simulink model "sl_aerialmanipulator"  (R2016b)
settings: Solver=FixedStepAuto  StartTime=0.0  StopTime=20  RelTol=1e-3
InitFcn:
  | % load a dynamic model of the quadrotor
  | mdl_aerialmanipulator
values from neighbouring files (symbols this model uses):
  ps = cam.project(Marker, 'Tcam', transl(CenterBias'+[0 0 TargetHeight])*trotx(-pi))    [mdl_aerialmanipulator.m]
undefined symbols (not defined in the file or in its folder): aerialmanipulator, rpy2tr, transl
undefined symbols (not defined in the file): manipulator
libraries: roblocks x6
settings Model: Creator=zhonghang  LastModifiedBy=dell
settings SolverCC: ZeroCrossControl=EnableAll
settings DataIOCC: LimitDataPoints=on  SaveFormat=Array
settings OptimizationCC: DefaultParameterBehavior=Inlined  UseDivisionForNetSlopeComputation=on  UseFloatMulNetSlope=on  InlineInvariantSignals=on  PassReuseOutputArgsAs=Individual arguments  ZeroExternalMemoryAtStartup=off  ZeroInternalMemoryAtStartup=off  NoFixptDivByZeroProtection=on  EfficientFloat2IntCast=on  LifeSpan=1
settings DebuggingCC: ParameterTunabilityLossMsg=error  SFUnexpectedBacktrackingDiag=warning  SFNoUnconditionalDefaultTransitionDiag=warning  SFExecutionAtInitializationDiag=none
settings ModelReferenceCC: PropagateSignalLabelsOutOfModel=off
settings RTWCC: SystemTargetFile=ert.tlc  TemplateMakefile=ert_default_tmf  Description=Embedded Coder  GenerateReport=on  IncludeHyperlinkInReport=on  LaunchReport=on  GenerateTraceInfo=on  GenerateTraceReport=on  GenerateTraceReportSl=on  GenerateTraceReportSf=on  GenerateTraceReportEml=on  GenerateCodeMetricsReport=on
settings CodeAppCC: ForceParamTrailComments=on  IgnoreCustomStorageClasses=off  OperatorAnnotations=on  SimulinkDataObjDesc=on  SFDataObjDesc=on  MATLABFcnDesc=on  CustomSymbolStrGlobalVar=rt$N$M  CustomSymbolStrType=$N$M  CustomSymbolStrFcn=$N$M$F  CustomSymbolStrMacro=$N$M  InsertBlockDesc=on  MATLABSourceComments=on
settings ERTTargetCC: GenerateSampleERTMain=on  CombineSignalStateStructs=on  SupportAbsoluteTime=off  SupportComplex=off  SupportContinuousTime=on  SupportNonInlinedSFcns=on  InlinedParameterPlacement=NonHierarchical  ERTCustomFileTemplate=example_file_process.tlc  ERTFilePackagingFormat=CompactWithDataFile
settings ConfigComp: CovMetricSettings=dw  CovHtmlReporting=on  CovSaveCumulativeToWorkspaceVar=on  CovSaveSingleToWorkspaceVar=on  CovExternalEMLEnable=off

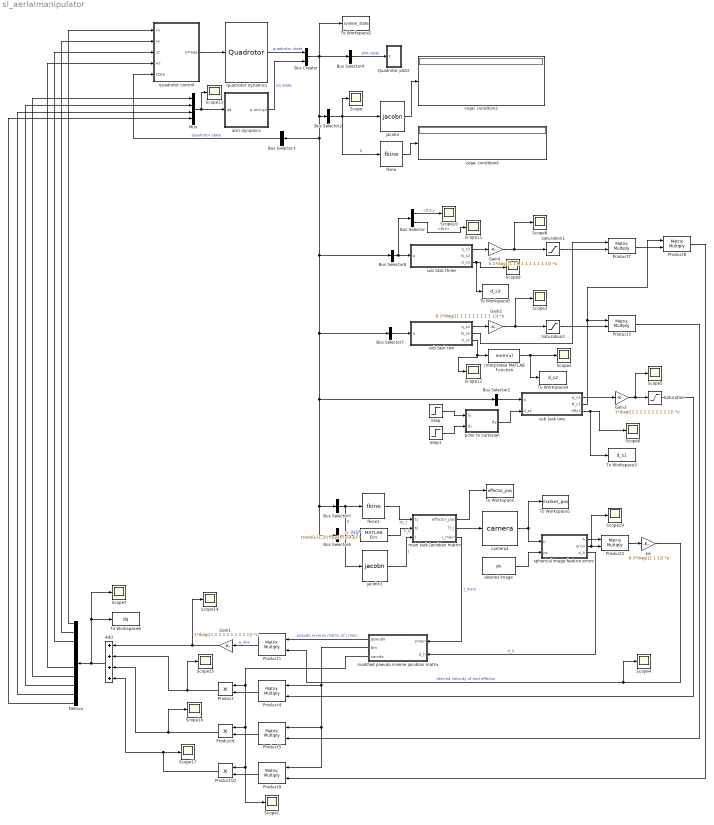
== system sl_aerialmanipulator ==
  -> SE2 : MATLABFcn  MATLABFcn=transl(u(1:3))*rpy2tr(u(4:6)')  OutputDimensions=[4 4]  Output1D=off
  Add : Sum  Inputs=++++
  Bus Creator : BusCreator  Inputs=2
  Bus Selector : BusSelector  OutputSignals=th1,th4
  Bus Selector1 : BusSelector  OutputSignals=quadrotor state.X,quadrotor state.Y,quadrotor state.Z,quadrotor state.roll,quadrotor state.pitch,quadrotor state.yaw,rm state.th1,rm state.th2,rm state.th3,rm state.th4  OutputAsBus=on
  Bus Selector{2,5,7..8} (4 alike) : BusSelector  OutputSignals=rm state.th1,rm state.th2,rm state.th3,rm state.th4  OutputAsBus=on
  Bus Selector3 : BusSelector  OutputSignals=quadrotor state.X,quadrotor state.Y,quadrotor state.Z,quadrotor state.yaw,quadrotor state.pitch,quadrotor state.roll,quadrotor state.dx,quadrotor state.dy,quadrotor state.dz,quadrotor state.dyaw,quadrotor state.dpitch,quadrotor state.droll  OutputAsBus=on
  Bus Selector4 : BusSelector  OutputSignals=quadrotor state.X,quadrotor state.Y,quadrotor state.Z,quadrotor state.yaw,quadrotor state.pitch,quadrotor state.roll,rm state.th1,rm state.th2,rm state.th3,rm state.th4  OutputAsBus=on
  Bus Selector6 : BusSelector  OutputSignals=quadrotor state.X,quadrotor state.Y,quadrotor state.Z,quadrotor state.yaw,quadrotor state.pitch,quadrotor state.roll  OutputAsBus=on
  Demux : Demux  Outputs=10
  Gain1 : Gain  Gain=1*diag([1 1 1 1 1 1 1 1 1 1])  Multiplication=Matrix(K*u)
  Gain2 : Gain  Gain=-0.1*diag([1 1 1 1 1 1 1 1 1 1])  Multiplication=Matrix(K*u)
  Gain3 : Gain  Gain=1*diag([1 1 1 1 1 1 1 1 1 1])  Multiplication=Matrix(K*u)
  Gain4 : Gain  Gain=0.1*diag([1 1 1 1 1 1 1 1 1 1])  Multiplication=Matrix(K*u)
  Interpreted MATLAB Function : MATLABFcn  MATLABFcn=norm(u)
  Mux : Mux
  Product : Product
  Product{1..5,7..9} (8 alike) : Product  Multiplication=Matrix(*)
  Product10 : Product
  Product6 : Product
  Quadrotor plot2 : Subsystem  AncestorBlock=roblocks/Robot Graphics/Quadrotor plot  mask{quad=aerialmanipulator, xydim=1.5, zdim=2.5}
      mask prompts: quad "Model"; xydim "xy-axes dimension"; zdim "z-axis dimension"
      mask help: Animate quadrotor.
      mask Help:
      | This block graphically displays a quadrotor (flying robot).
      | 
      | A new figure is created and A graphical model of a quadrotor is animated
      | to a pose specified by the state vector input to the block.
      | 
      | The state vector is [x y z roll pitch yaw] in world coordinates and the
      | angles are in radians.
      | 
      | Notes:
      | - The dimensions of the vehicle workspace are set by parameters
  Saturation : Saturate  UpperLimit=1  LowerLimit=-1
  Saturation1 : Saturate  UpperLimit=1  LowerLimit=-1
  Saturation2 : Saturate  UpperLimit=1  LowerLimit=-1
  Scope{,1..17,19} (19 alike) : Scope
  Step : Step  Time=15  Before=180*pi/180  After=120*pi/180  SampleTime=0
  Step1 : Step  Time=15  Before=0*pi/180  After=-120*pi/180  SampleTime=0
  To Workspace : ToWorkspace  VariableName=effector_pos  SaveFormat=Structure With Time  SampleTime=-1
  To Workspace1 : ToWorkspace  VariableName=marker_pos  SaveFormat=Structure With Time  SampleTime=-1
  To Workspace2 : ToWorkspace  VariableName=system_state  SaveFormat=Structure With Time  SampleTime=-1
  To Workspace3 : ToWorkspace  VariableName=d_s1  SaveFormat=Structure With Time  SampleTime=-1
  To Workspace4 : ToWorkspace  VariableName=d_s2  SaveFormat=Structure With Time  SampleTime=-1
  To Workspace5 : ToWorkspace  VariableName=d_s3  SaveFormat=Structure With Time  SampleTime=-1
  To Workspace6 : ToWorkspace  VariableName=dq  SaveFormat=Structure With Time  SampleTime=-1
  arm dynamics : Subsystem  mask{robotarm=manipulator, q0=[-pi/3 3*pi/4 0 0]}
      mask prompts: robotarm "robot arm object"; q0 "joint initial value"
  camera2 : roblocks/Vision/camera  cam=cam  points=Marker
  desired image : Constant  Value=ps  VectorParams1D=off
  fkine : roblocks/Kinematics/fkine  robot=manipulator
  fkine1 : roblocks/Kinematics/fkine  robot=manipulator
  jacobn : roblocks/Kinematics/jacobn  robot=manipulator
  jacobn1 : roblocks/Kinematics/jacobn  robot=manipulator
  kd : Gain  Gain=0.3*diag([1 1 1])  Multiplication=Matrix(K*u)
  main task Jacobian matrix : MATLAB Function  TreatAsAtomicUnit=on
  modified pseudo inverse jacobian matrix : MATLAB Function  TreatAsAtomicUnit=on
  polor to cartesian : MATLAB Function  TreatAsAtomicUnit=on
  quadrotor control : Subsystem
  quadrotor dynamics : roblocks/Dynamics/Quadrotor  quad=aerialmanipulator
      link override Dynamics: FunctionName=aerialmanipulator_dynamics
  "spherical image feature errors " : MATLAB Function  TreatAsAtomicUnit=on
  sub task one : MATLAB Function  TreatAsAtomicUnit=on
  sub task three : MATLAB Function  TreatAsAtomicUnit=on
  sub task two : MATLAB Function  TreatAsAtomicUnit=on
  visjac condition2 : Display
  visjac condition6 : Display
  wires:
  quadrotor control/1(omega) -> quadrotor dynamics/1
  quadrotor dynamics/1 -> Bus Creator/1  "quadrotor state"
  jacobn/1 -> visjac condition2/1
  Bus Selector2/1 -> Scope/1, fkine/1, jacobn/1  "q"
  Bus Selector3/1 -> quadrotor control/5(state)  "quadrotor state"
  Bus Selector4/1 -> Quadrotor plot2/1(X)  "plot state"
  fkine/1 -> visjac condition6/1
  Bus Selector5/1 -> jacobn1/1, fkine1/1  "q"
  Bus Selector6/1 -> -> SE2/1  "quad"
  fkine1/1 -> main task Jacobian matrix/1(t1)  "Tb_t"
  -> SE2/1 -> main task Jacobian matrix/2(t2)  "Ti_b"
  jacobn1/1 -> main task Jacobian matrix/3(J)  "J"
  Product1/1 -> Gain1/1  "q_des"
  "spherical image feature errors "/1(A) -> Product2/1
  Product2/1 -> kd/1
  "spherical image feature errors "/2(error) -> Scope19/1, Product2/2
  "spherical image feature errors "/3(d_h) -> modified pseudo inverse jacobian matrix/2(d_h)  "d_h"
  modified pseudo inverse jacobian matrix/1(Jpseudo) -> Product1/1  "pseudo inverse matrix of J main"
  Bus Selector1/1 -> sub task one/1(q)
  sub task one/1(q_s1) -> Gain3/1
  modified pseudo inverse jacobian matrix/2(Nm) -> Product9/1, Product5/1, Product4/1
  camera2/1 -> "spherical image feature errors "/1(p), To Workspace1/1
  Bus Creator/1 -> To Workspace2/1, Bus Selector3/1, Bus Selector6/1, Bus Selector5/1, Bus Selector1/1, Bus Selector7/1, Bus Selector8/1, Bus Selector2/1, Bus Selector4/1
  Bus Selector7/1 -> sub task two/1(q)
  sub task two/1(q_s2) -> Gain2/1
  Interpreted MATLAB Function/1 -> To Workspace4/1, Scope2/1
  sub task two/3(d_s2) -> Scope12/1, Interpreted MATLAB Function/1
  kd/1 -> Scope4/1, Product1/2  "desired velocity of end effector"
  Gain2/1 -> Saturation2/1, Scope3/1
  sub task one/2(N_s1) -> Product8/1, Product3/1
  Gain3/1 -> Saturation/1, Scope5/1
  Product4/1 -> Product/2
  Product5/1 -> Product6/2
  Bus Selector8/1 -> Bus Selector/1, sub task three/1(q)
  sub task three/1(q_s3) -> Gain4/1
  Gain4/1 -> Saturation1/1, Scope8/1
  Product9/1 -> Product10/2
  sub task three/3(d_s3) -> To Workspace5/1, Scope9/1
  Bus Selector/1 -> Scope10/1  "<th1>"
  Bus Selector/2 -> Scope11/1  "<th4>"
  Gain1/1 -> Scope14/1, Add/1
  Add/1 -> To Workspace6/1, Scope7/1, Demux/1
  Demux/1 -> quadrotor control/1(vx)
  Demux/2 -> quadrotor control/2(vy)
  Demux/3 -> quadrotor control/3(vz)
  Demux/7 -> Mux/1
  Demux/8 -> Mux/2
  Demux/9 -> Mux/3
  main task Jacobian matrix/2(Tt_i) -> camera2/1
  main task Jacobian matrix/3(J_main) -> modified pseudo inverse jacobian matrix/1(Jmain)  "J_main"
  modified pseudo inverse jacobian matrix/3(namda) -> Product6/1, Product10/1, Scope1/1, Product/1
  desired image/1 -> "spherical image feature errors "/2(ps)
  polor to cartesian/1(dy) -> sub task one/2(d_s1)
  Step/1 -> polor to cartesian/1(fy)
  Step1/1 -> polor to cartesian/2(th)
  main task Jacobian matrix/1(effector_pos) -> To Workspace/1
  Saturation2/1 -> Product3/2
  sub task two/2(N_s2) -> Product7/1
  Product7/1 -> Product8/2
  Product/1 -> Add/2, Scope15/1
  Product6/1 -> Add/3, Scope16/1
  Saturation1/1 -> Product7/2
  Product10/1 -> Add/4, Scope17/1
  Saturation/1 -> Product4/2
  Product3/1 -> Product5/2
  Product8/1 -> Product9/2
  sub task one/3(dRs1) -> To Workspace3/1, Scope6/1
  Mux/1 -> Scope13/1, arm dynamics/1(qd)
  arm dynamics/1(q and qd) -> Bus Creator/2  "rm state"
  Demux/6 -> quadrotor control/4(wz)
  Demux/10 -> Mux/4

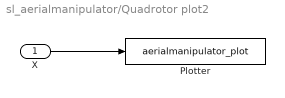
== system sl_aerialmanipulator/Quadrotor plot2 ==
  X : Inport
  Plotter : S-Function  FunctionName=aerialmanipulator_plot  Parameters=[xydim, zdim], 1, 1,aerialmanipulator  SFunctionDeploymentMode=off  EnableBusSupport=off
  wires:
  X/1 -> Plotter/1

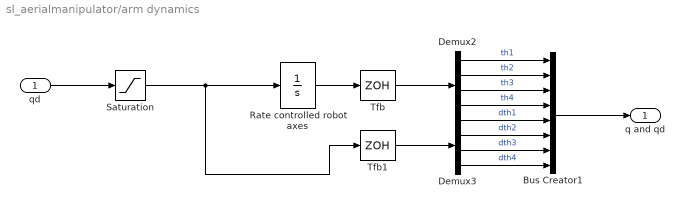
== system sl_aerialmanipulator/arm dynamics ==
  qd : Inport
  Bus Creator1 : BusCreator  Inputs=8
  Demux2 : Demux
  Demux3 : Demux
  Rate controlled robot axes : Integrator  InitialCondition=q0
  Saturation : Saturate  UpperLimit=1  LowerLimit=-1
  Tfb : ZeroOrderHold  SampleTime=0.01
  Tfb1 : ZeroOrderHold  SampleTime=0.01
  q and qd : Outport
  wires:
  qd/1 -> Saturation/1
  Rate controlled robot axes/1 -> Tfb/1
  Demux3/4 -> Bus Creator1/8  "dth4"
  Demux3/3 -> Bus Creator1/7  "dth3"
  Demux3/2 -> Bus Creator1/6  "dth2"
  Demux3/1 -> Bus Creator1/5  "dth1"
  Demux2/4 -> Bus Creator1/4  "th4"
  Demux2/3 -> Bus Creator1/3  "th3"
  Demux2/2 -> Bus Creator1/2  "th2"
  Demux2/1 -> Bus Creator1/1  "th1"
  Bus Creator1/1 -> q and qd/1
  Saturation/1 -> Tfb1/1, Rate controlled robot axes/1
  Tfb/1 -> Demux2/1
  Tfb1/1 -> Demux3/1

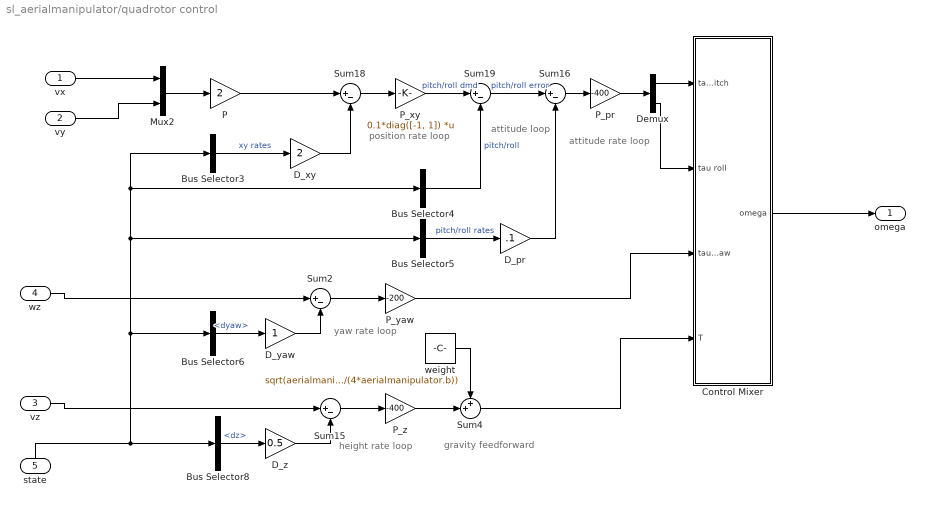
== system sl_aerialmanipulator/quadrotor control ==
  note: gravity feedforward
  note: attitude rate
      | loop
  note: attitude
      | loop
  note: position rate
      | loop
  note: yaw rate
      | loop
  note: height rate
      | loop
  vx : Inport
  vy : Inport  Port=2
  vz : Inport  Port=3
  wz : Inport  Port=4
  state : Inport  Port=5
  Bus Selector3 : BusSelector  OutputSignals=dx,dy  OutputAsBus=on
  Bus Selector4 : BusSelector  OutputSignals=pitch,roll  OutputAsBus=on
  Bus Selector5 : BusSelector  OutputSignals=dpitch,droll  OutputAsBus=on
  Bus Selector6 : BusSelector  OutputSignals=dyaw
  Bus Selector8 : BusSelector  OutputSignals=dz
  Control Mixer : Subsystem  AncestorBlock=roblocks/Dynamics/Control Mixer 4
      mask help: Quadrotor control mixer
      mask Help:
      | Determine rotor speeds based on desired torques and thrust.
      | 
      | <b>Inputs::</b>
      | 
      | tau pitch (1x1)  desired pitching torque [Nm]
      | tau roll (1x1)   desired rolling torque [Nm]
      | tau yaw (1x1)    desired yawing torque [Nm]
      | T (1x1)          desired thrust [N]
      | 
      | <b>Outputs::</b>
      | 
      | w1 (1x1) angular velocity of rotor 1 [rad]
      | w2 (1x1) angular velocity of rotor 2 [rad]
      | w3 (1x1) angular velocity of rotor 3 [rad]
      | w4 (1x1) angular velocity of rotor 4 [rad]
      | 
      | <b>Notes::</b>
      | 
      | - Assumes the rotor labelling convention of RVC Fig 4.16.
      | - The quadrotor is underactuated and has only 4 inputs.
  D_pr : Gain  Gain=.1
  D_xy : Gain  Gain=2
  D_yaw : Gain
  D_z : Gain  Gain=0.5
  Demux : Demux  Outputs=2
  Mux2 : Mux  Inputs=2
  P : Gain  Gain=2
  P_pr : Gain  Gain=-400
  P_xy : Gain  Gain=0.1*diag([-1, 1])  Multiplication=Matrix(K*u)
  P_yaw : Gain  Gain=-200
  P_z : Gain  Gain=-400
  Sum{2,15..16,18..19} (5 alike) : Sum  Inputs=|+-
  Sum4 : Sum  Inputs=++|
  weight : Constant  Value=sqrt(aerialmanipulator.M*aerialmanipulator.g/(4*aerialmanipulator.b))  SampleTime=0
  omega : Outport
  wires:
  state/1 -> Bus Selector8/1, Bus Selector5/1, Bus Selector4/1, Bus Selector3/1, Bus Selector6/1
  Mux2/1 -> P/1
  P/1 -> Sum18/1
  Sum18/1 -> P_xy/1
  wz/1 -> Sum2/1
  vz/1 -> Sum15/1
  Control Mixer/1(omega) -> omega/1
  Bus Selector3/1 -> D_xy/1  "xy rates"
  D_xy/1 -> Sum18/2
  P_xy/1 -> Sum19/1  "pitch/roll dmd"
  Bus Selector4/1 -> Sum19/2  "pitch/roll"
  Sum19/1 -> Sum16/1  "pitch/roll error"
  P_pr/1 -> Demux/1
  Bus Selector6/1 -> D_yaw/1  "<dyaw>"
  Bus Selector8/1 -> D_z/1  "<dz>"
  D_z/1 -> Sum15/2
  D_pr/1 -> Sum16/2
  Demux/2 -> Control Mixer/2(tau roll)
  Sum2/1 -> P_yaw/1
  P_yaw/1 -> Control Mixer/3(tau yaw)
  Demux/1 -> Control Mixer/1(tau pitch)
  Bus Selector5/1 -> D_pr/1  "pitch/roll rates"
  D_yaw/1 -> Sum2/2
  weight/1 -> Sum4/1
  Sum4/1 -> Control Mixer/4(T)
  vx/1 -> Mux2/1
  Sum16/1 -> P_pr/1
  vy/1 -> Mux2/2
  Sum15/1 -> P_z/1
  P_z/1 -> Sum4/2

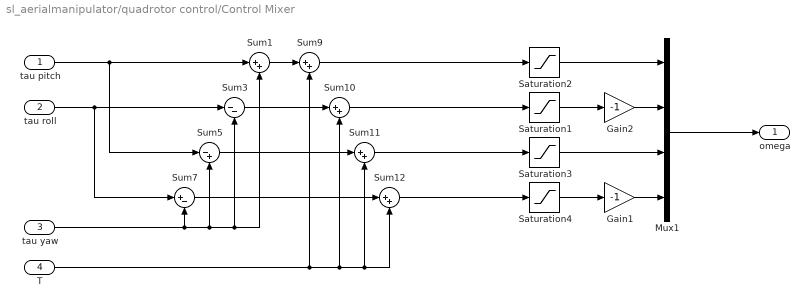
== system sl_aerialmanipulator/quadrotor control/Control Mixer ==
  tau pitch : Inport
  tau roll : Inport  Port=2
  tau yaw : Inport  Port=3
  T : Inport  Port=4
  Gain1 : Gain  Gain=-1
  Gain2 : Gain  Gain=-1
  Mux1 : Mux
  Saturation{1..4} (4 alike) : Saturate  UpperLimit=1000  LowerLimit=700
  Sum{1,9..12} (5 alike) : Sum  Inputs=|++  SaturateOnIntegerOverflow=on  InputSameDT=on  OutDataTypeStr=Inherit: Same as first input
  Sum3 : Sum  Inputs=|--  SaturateOnIntegerOverflow=on  InputSameDT=on  OutDataTypeStr=Inherit: Same as first input
  Sum5 : Sum  Inputs=|-+  SaturateOnIntegerOverflow=on  InputSameDT=on  OutDataTypeStr=Inherit: Same as first input
  Sum7 : Sum  Inputs=|+-  SaturateOnIntegerOverflow=on  InputSameDT=on  OutDataTypeStr=Inherit: Same as first input
  omega : Outport
  wires:
  Mux1/1 -> omega/1
  Gain2/1 -> Mux1/2
  tau yaw/1 -> Sum7/2, Sum5/2, Sum3/2, Sum1/2
  Saturation2/1 -> Mux1/1
  Saturation1/1 -> Gain2/1
  Saturation3/1 -> Mux1/3
  Saturation4/1 -> Gain1/1
  tau pitch/1 -> Sum1/1, Sum5/1
  Sum1/1 -> Sum9/1
  Sum3/1 -> Sum10/1
  Sum5/1 -> Sum11/1
  Sum7/1 -> Sum12/1
  Sum9/1 -> Saturation2/1
  Sum10/1 -> Saturation1/1
  Sum11/1 -> Saturation3/1
  Sum12/1 -> Saturation4/1
  T/1 -> Sum11/2, Sum12/2, Sum10/2, Sum9/2
  tau roll/1 -> Sum3/1, Sum7/1
  Gain1/1 -> Mux1/4

== matlab function sl_aerialmanipulator/main task Jacobian matrix ==
  data: effector_pos output; Tt_i output; t1 input; J_main output; t2 input; J input
function [effector_pos, Tt_i,J_main] = JmainCal(t1, t2, J)
%#codegen

Base_T =[0.7071 0.7071 0 0; ...
    -0.7071 0.7071 0 0; ...
    0 0 -1.0000 0; ...
    0 0 0 1.0000];
s = t2*Base_T*t1;
s1 = s(1:3, 1:3);
% transfer end effevtor to interial coor matrix 
Tt_i = s;
% end effector position
effector_pos = s(1:3,4)';
% R is tthe R_I_T
R = pinv(s1);
% J_l
Jl = J(1:3, :);
% J main task jacobian matrix
J_main = [R zeros(3) Jl];

== matlab function sl_aerialmanipulator/sub task one ==
  data: q_s1 output; N_s1 output; q input; d_s1 input; dRs1 output
function [q_s1, N_s1, dRs1] = SubTskOneJaco(q, d_s1)
%#codegen
%%
x = zeros(10,1);
x = q;
roll = x(4); pitch = x(5); yaw = x(6);
th1 = x(7); th2 = x(8); th3 = x(9); th4 = x(10);
%% jacobian matrix
d_Rs1 = [0, 0, 0, 0, 0, 0,                                                                                                         ((7071*cos(pitch))/10000 + (7071*sin(pitch)*sin(roll))/10000)*((4967757600021511*sin(th1))/81129638414606681695789005144064 + cos(th3)*(cos(th1)*cos(th2) - (4967757600021511*sin(th1)*sin(th2))/81129638414606681695789005144064) - sin(th3)*(cos(th1)*sin(th2) + (4967757600021511*cos(th2)*sin(th1))/81129638414606681695789005144064)) - ((7071*cos(pitch))/10000 - (7071*sin(pitch)*sin(roll))/10000)*(cos(th3)*((4967757600021511*cos(th1)*sin(th2))/81129638414606681695789005144064 + cos(th2)*sin(th1)) - (4967757600021511*cos(th1))/81129638414606681695789005144064 + sin(th3)*((4967757600021511*cos(th1)*cos(th2))/81129638414606681695789005144064 - sin(th1)*sin(th2))),                                                                                                                                         (cos(th3)*((4967757600021511*cos(th1)*cos(th2))/81129638414606681695789005144064 - sin(th1)*sin(th2)) - sin(th3)*((4967757600021511*cos(th1)*sin(th2))/81129638414606681695789005144064 + cos(th2)*sin(th1)))*((7071*cos(pitch))/10000 + (7071*sin(pitch)*sin(roll))/10000) - (cos(th3)*(cos(th1)*sin(th2) + (4967757600021511*cos(th2)*sin(th1))/81129638414606681695789005144064) + sin(th3)*(cos(th1)*cos(th2) - (4967757600021511*sin(th1)*sin(th2))/81129638414606681695789005144064))*((7071*cos(pitch))/10000 - (7071*sin(pitch)*sin(roll))/10000) - cos(roll)*sin(pitch)*(cos(th2)*cos(th3) - sin(th2)*sin(th3)),                                                                                                                                         (cos(th3)*((4967757600021511*cos(th1)*cos(th2))/81129638414606681695789005144064 - sin(th1)*sin(th2)) - sin(th3)*((4967757600021511*cos(th1)*sin(th2))/81129638414606681695789005144064 + cos(th2)*sin(th1)))*((7071*cos(pitch))/10000 + (7071*sin(pitch)*sin(roll))/10000) - (cos(th3)*(cos(th1)*sin(th2) + (4967757600021511*cos(th2)*sin(th1))/81129638414606681695789005144064) + sin(th3)*(cos(th1)*cos(th2) - (4967757600021511*sin(th1)*sin(th2))/81129638414606681695789005144064))*((7071*cos(pitch))/10000 - (7071*sin(pitch)*sin(roll))/10000) - cos(roll)*sin(pitch)*(cos(th2)*cos(th3) - sin(th2)*sin(th3)), 0; ...
    0, 0, 0, 0, 0, 0, ((7071*cos(roll)*cos(yaw))/10000 + (7071*sin(pitch)*sin(yaw))/10000 - (7071*cos(pitch)*sin(roll)*sin(yaw))/10000)*((4967757600021511*sin(th1))/81129638414606681695789005144064 + cos(th3)*(cos(th1)*cos(th2) - (4967757600021511*sin(th1)*sin(th2))/81129638414606681695789005144064) - sin(th3)*(cos(th1)*sin(th2) + (4967757600021511*cos(th2)*sin(th1))/81129638414606681695789005144064)) - ((7071*sin(pitch)*sin(yaw))/10000 - (7071*cos(roll)*cos(yaw))/10000 + (7071*cos(pitch)*sin(roll)*sin(yaw))/10000)*(cos(th3)*((4967757600021511*cos(th1)*sin(th2))/81129638414606681695789005144064 + cos(th2)*sin(th1)) - (4967757600021511*cos(th1))/81129638414606681695789005144064 + sin(th3)*((4967757600021511*cos(th1)*cos(th2))/81129638414606681695789005144064 - sin(th1)*sin(th2))), (cos(yaw)*sin(roll) + cos(pitch)*cos(roll)*sin(yaw))*(cos(th2)*cos(th3) - sin(th2)*sin(th3)) - (cos(th3)*(cos(th1)*sin(th2) + (4967757600021511*cos(th2)*sin(th1))/81129638414606681695789005144064) + sin(th3)*(cos(th1)*cos(th2) - (4967757600021511*sin(th1)*sin(th2))/81129638414606681695789005144064))*((7071*sin(pitch)*sin(yaw))/10000 - (7071*cos(roll)*cos(yaw))/10000 + (7071*cos(pitch)*sin(roll)*sin(yaw))/10000) + (cos(th3)*((4967757600021511*cos(th1)*cos(th2))/81129638414606681695789005144064 - sin(th1)*sin(th2)) - sin(th3)*((4967757600021511*cos(th1)*sin(th2))/81129638414606681695789005144064 + cos(th2)*sin(th1)))*((7071*cos(roll)*cos(yaw))/10000 + (7071*sin(pitch)*sin(yaw))/10000 - (7071*cos(pitch)*sin(roll)*sin(yaw))/10000), (cos(yaw)*sin(roll) + cos(pitch)*cos(roll)*sin(yaw))*(cos(th2)*cos(th3) - sin(th2)*sin(th3)) - (cos(th3)*(cos(th1)*sin(th2) + (4967757600021511*cos(th2)*sin(th1))/81129638414606681695789005144064) + sin(th3)*(cos(th1)*cos(th2) - (4967757600021511*sin(th1)*sin(th2))/81129638414606681695789005144064))*((7071*sin(pitch)*sin(yaw))/10000 - (7071*cos(roll)*cos(yaw))/10000 + (7071*cos(pitch)*sin(roll)*sin(yaw))/10000) + (cos(th3)*((4967757600021511*cos(th1)*cos(th2))/81129638414606681695789005144064 - sin(th1)*sin(th2)) - sin(th3)*((4967757600021511*cos(th1)*sin(th2))/81129638414606681695789005144064 + cos(th2)*sin(th1)))*((7071*cos(roll)*cos(yaw))/10000 + (7071*sin(pitch)*sin(yaw))/10000 - (7071*cos(pitch)*sin(roll)*sin(yaw))/10000), 0; ...
    0, 0, 0, 0, 0, 0, ((7071*cos(yaw)*sin(pitch))/10000 + (7071*cos(roll)*sin(yaw))/10000 + (7071*cos(pitch)*cos(yaw)*sin(roll))/10000)*(cos(th3)*((4967757600021511*cos(th1)*sin(th2))/81129638414606681695789005144064 + cos(th2)*sin(th1)) - (4967757600021511*cos(th1))/81129638414606681695789005144064 + sin(th3)*((4967757600021511*cos(th1)*cos(th2))/81129638414606681695789005144064 - sin(th1)*sin(th2))) + ((7071*cos(roll)*sin(yaw))/10000 - (7071*cos(yaw)*sin(pitch))/10000 + (7071*cos(pitch)*cos(yaw)*sin(roll))/10000)*((4967757600021511*sin(th1))/81129638414606681695789005144064 + cos(th3)*(cos(th1)*cos(th2) - (4967757600021511*sin(th1)*sin(th2))/81129638414606681695789005144064) - sin(th3)*(cos(th1)*sin(th2) + (4967757600021511*cos(th2)*sin(th1))/81129638414606681695789005144064)), (sin(roll)*sin(yaw) - cos(pitch)*cos(roll)*cos(yaw))*(cos(th2)*cos(th3) - sin(th2)*sin(th3)) + (cos(th3)*(cos(th1)*sin(th2) + (4967757600021511*cos(th2)*sin(th1))/81129638414606681695789005144064) + sin(th3)*(cos(th1)*cos(th2) - (4967757600021511*sin(th1)*sin(th2))/81129638414606681695789005144064))*((7071*cos(yaw)*sin(pitch))/10000 + (7071*cos(roll)*sin(yaw))/10000 + (7071*cos(pitch)*cos(yaw)*sin(roll))/10000) + (cos(th3)*((4967757600021511*cos(th1)*cos(th2))/81129638414606681695789005144064 - sin(th1)*sin(th2)) - sin(th3)*((4967757600021511*cos(th1)*sin(th2))/81129638414606681695789005144064 + cos(th2)*sin(th1)))*((7071*cos(roll)*sin(yaw))/10000 - (7071*cos(yaw)*sin(pitch))/10000 + (7071*cos(pitch)*cos(yaw)*sin(roll))/10000), (sin(roll)*sin(yaw) - cos(pitch)*cos(roll)*cos(yaw))*(cos(th2)*cos(th3) - sin(th2)*sin(th3)) + (cos(th3)*(cos(th1)*sin(th2) + (4967757600021511*cos(th2)*sin(th1))/81129638414606681695789005144064) + sin(th3)*(cos(th1)*cos(th2) - (4967757600021511*sin(th1)*sin(th2))/81129638414606681695789005144064))*((7071*cos(yaw)*sin(pitch))/10000 + (7071*cos(roll)*sin(yaw))/10000 + (7071*cos(pitch)*cos(yaw)*sin(roll))/10000) + (cos(th3)*((4967757600021511*cos(th1)*cos(th2))/81129638414606681695789005144064 - sin(th1)*sin(th2)) - sin(th3)*((4967757600021511*cos(th1)*sin(th2))/81129638414606681695789005144064 + cos(th2)*sin(th1)))*((7071*cos(roll)*sin(yaw))/10000 - (7071*cos(yaw)*sin(pitch))/10000 + (7071*cos(pitch)*cos(yaw)*sin(roll))/10000), 0];
%d_Rs1 = [0, 0, 0,                                                                                                                           (7071*cos(roll)*sin(pitch)*(cos(th3)*((4967757600021511*cos(th1)*sin(th2))/81129638414606681695789005144064 + cos(th2)*sin(th1)) - (4967757600021511*cos(th1))/81129638414606681695789005144064 + sin(th3)*((4967757600021511*cos(th1)*cos(th2))/81129638414606681695789005144064 - sin(th1)*sin(th2))))/10000 - (7071*cos(roll)*sin(pitch)*((4967757600021511*sin(th1))/81129638414606681695789005144064 + cos(th3)*(cos(th1)*cos(th2) - (4967757600021511*sin(th1)*sin(th2))/81129638414606681695789005144064) - sin(th3)*(cos(th1)*sin(th2) + (4967757600021511*cos(th2)*sin(th1))/81129638414606681695789005144064)))/10000 + sin(pitch)*sin(roll)*(cos(th2)*sin(th3) + cos(th3)*sin(th2) + 24678615572571482867467662723121/6582018229284824168619876730229402019930943462534319453394436096),                                            - ((7071*sin(pitch))/10000 - (7071*cos(pitch)*sin(roll))/10000)*(cos(th3)*((4967757600021511*cos(th1)*sin(th2))/81129638414606681695789005144064 + cos(th2)*sin(th1)) - (4967757600021511*cos(th1))/81129638414606681695789005144064 + sin(th3)*((4967757600021511*cos(th1)*cos(th2))/81129638414606681695789005144064 - sin(th1)*sin(th2))) - ((7071*sin(pitch))/10000 + (7071*cos(pitch)*sin(roll))/10000)*((4967757600021511*sin(th1))/81129638414606681695789005144064 + cos(th3)*(cos(th1)*cos(th2) - (4967757600021511*sin(th1)*sin(th2))/81129638414606681695789005144064) - sin(th3)*(cos(th1)*sin(th2) + (4967757600021511*cos(th2)*sin(th1))/81129638414606681695789005144064)) - cos(pitch)*cos(roll)*(cos(th2)*sin(th3) + cos(th3)*sin(th2) + 24678615572571482867467662723121/6582018229284824168619876730229402019930943462534319453394436096),                                                                                                                                                                                                                                                                                                                                                                                                                                                                                                                                                                                                                                                                                                                                                                                                                                                                                                                                                                                                  0,                                                                                                         ((7071*cos(pitch))/10000 + (7071*sin(pitch)*sin(roll))/10000)*((4967757600021511*sin(th1))/81129638414606681695789005144064 + cos(th3)*(cos(th1)*cos(th2) - (4967757600021511*sin(th1)*sin(th2))/81129638414606681695789005144064) - sin(th3)*(cos(th1)*sin(th2) + (4967757600021511*cos(th2)*sin(th1))/81129638414606681695789005144064)) - ((7071*cos(pitch))/10000 - (7071*sin(pitch)*sin(roll))/10000)*(cos(th3)*((4967757600021511*cos(th1)*sin(th2))/81129638414606681695789005144064 + cos(th2)*sin(th1)) - (4967757600021511*cos(th1))/81129638414606681695789005144064 + sin(th3)*((4967757600021511*cos(th1)*cos(th2))/81129638414606681695789005144064 - sin(th1)*sin(th2))),                                                                                                                                         (cos(th3)*((4967757600021511*cos(th1)*cos(th2))/81129638414606681695789005144064 - sin(th1)*sin(th2)) - sin(th3)*((4967757600021511*cos(th1)*sin(th2))/81129638414606681695789005144064 + cos(th2)*sin(th1)))*((7071*cos(pitch))/10000 + (7071*sin(pitch)*sin(roll))/10000) - (cos(th3)*(cos(th1)*sin(th2) + (4967757600021511*cos(th2)*sin(th1))/81129638414606681695789005144064) + sin(th3)*(cos(th1)*cos(th2) - (4967757600021511*sin(th1)*sin(th2))/81129638414606681695789005144064))*((7071*cos(pitch))/10000 - (7071*sin(pitch)*sin(roll))/10000) - cos(roll)*sin(pitch)*(cos(th2)*cos(th3) - sin(th2)*sin(th3)),                                                                                                                                         (cos(th3)*((4967757600021511*cos(th1)*cos(th2))/81129638414606681695789005144064 - sin(th1)*sin(th2)) - sin(th3)*((4967757600021511*cos(th1)*sin(th2))/81129638414606681695789005144064 + cos(th2)*sin(th1)))*((7071*cos(pitch))/10000 + (7071*sin(pitch)*sin(roll))/10000) - (cos(th3)*(cos(th1)*sin(th2) + (4967757600021511*cos(th2)*sin(th1))/81129638414606681695789005144064) + sin(th3)*(cos(th1)*cos(th2) - (4967757600021511*sin(th1)*sin(th2))/81129638414606681695789005144064))*((7071*cos(pitch))/10000 - (7071*sin(pitch)*sin(roll))/10000) - cos(roll)*sin(pitch)*(cos(th2)*cos(th3) - sin(th2)*sin(th3)), 0; ...
%  0, 0, 0, (cos(roll)*cos(yaw) - cos(pitch)*sin(roll)*sin(yaw))*(cos(th2)*sin(th3) + cos(th3)*sin(th2) + 24678615572571482867467662723121/6582018229284824168619876730229402019930943462534319453394436096) - ((7071*cos(yaw)*sin(roll))/10000 + (7071*cos(pitch)*cos(roll)*sin(yaw))/10000)*(cos(th3)*((4967757600021511*cos(th1)*sin(th2))/81129638414606681695789005144064 + cos(th2)*sin(th1)) - (4967757600021511*cos(th1))/81129638414606681695789005144064 + sin(th3)*((4967757600021511*cos(th1)*cos(th2))/81129638414606681695789005144064 - sin(th1)*sin(th2))) + ((7071*cos(yaw)*sin(roll))/10000 + (7071*cos(pitch)*cos(roll)*sin(yaw))/10000)*((4967757600021511*sin(th1))/81129638414606681695789005144064 + cos(th3)*(cos(th1)*cos(th2) - (4967757600021511*sin(th1)*sin(th2))/81129638414606681695789005144064) - sin(th3)*(cos(th1)*sin(th2) + (4967757600021511*cos(th2)*sin(th1))/81129638414606681695789005144064)), ((7071*cos(pitch)*sin(yaw))/10000 + (7071*sin(pitch)*sin(roll)*sin(yaw))/10000)*(cos(th3)*((4967757600021511*cos(th1)*sin(th2))/81129638414606681695789005144064 + cos(th2)*sin(th1)) - (4967757600021511*cos(th1))/81129638414606681695789005144064 + sin(th3)*((4967757600021511*cos(th1)*cos(th2))/81129638414606681695789005144064 - sin(th1)*sin(th2))) + ((7071*cos(pitch)*sin(yaw))/10000 - (7071*sin(pitch)*sin(roll)*sin(yaw))/10000)*((4967757600021511*sin(th1))/81129638414606681695789005144064 + cos(th3)*(cos(th1)*cos(th2) - (4967757600021511*sin(th1)*sin(th2))/81129638414606681695789005144064) - sin(th3)*(cos(th1)*sin(th2) + (4967757600021511*cos(th2)*sin(th1))/81129638414606681695789005144064)) - cos(roll)*sin(pitch)*sin(yaw)*(cos(th2)*sin(th3) + cos(th3)*sin(th2) + 24678615572571482867467662723121/6582018229284824168619876730229402019930943462534319453394436096), ((7071*cos(yaw)*sin(pitch))/10000 + (7071*cos(roll)*sin(yaw))/10000 + (7071*cos(pitch)*cos(yaw)*sin(roll))/10000)*((4967757600021511*sin(th1))/81129638414606681695789005144064 + cos(th3)*(cos(th1)*cos(th2) - (4967757600021511*sin(th1)*sin(th2))/81129638414606681695789005144064) - sin(th3)*(cos(th1)*sin(th2) + (4967757600021511*cos(th2)*sin(th1))/81129638414606681695789005144064)) - ((7071*cos(roll)*sin(yaw))/10000 - (7071*cos(yaw)*sin(pitch))/10000 + (7071*cos(pitch)*cos(yaw)*sin(roll))/10000)*(cos(th3)*((4967757600021511*cos(th1)*sin(th2))/81129638414606681695789005144064 + cos(th2)*sin(th1)) - (4967757600021511*cos(th1))/81129638414606681695789005144064 + sin(th3)*((4967757600021511*cos(th1)*cos(th2))/81129638414606681695789005144064 - sin(th1)*sin(th2))) - (sin(roll)*sin(yaw) - cos(pitch)*cos(roll)*cos(yaw))*(cos(th2)*sin(th3) + cos(th3)*sin(th2) + 24678615572571482867467662723121/6582018229284824168619876730229402019930943462534319453394436096), ((7071*cos(roll)*cos(yaw))/10000 + (7071*sin(pitch)*sin(yaw))/10000 - (7071*cos(pitch)*sin(roll)*sin(yaw))/10000)*((4967757600021511*sin(th1))/81129638414606681695789005144064 + cos(th3)*(cos(th1)*cos(th2) - (4967757600021511*sin(th1)*sin(th2))/81129638414606681695789005144064) - sin(th3)*(cos(th1)*sin(th2) + (4967757600021511*cos(th2)*sin(th1))/81129638414606681695789005144064)) - ((7071*sin(pitch)*sin(yaw))/10000 - (7071*cos(roll)*cos(yaw))/10000 + (7071*cos(pitch)*sin(roll)*sin(yaw))/10000)*(cos(th3)*((4967757600021511*cos(th1)*sin(th2))/81129638414606681695789005144064 + cos(th2)*sin(th1)) - (4967757600021511*cos(th1))/81129638414606681695789005144064 + sin(th3)*((4967757600021511*cos(th1)*cos(th2))/81129638414606681695789005144064 - sin(th1)*sin(th2))), (cos(yaw)*sin(roll) + cos(pitch)*cos(roll)*sin(yaw))*(cos(th2)*cos(th3) - sin(th2)*sin(th3)) - (cos(th3)*(cos(th1)*sin(th2) + (4967757600021511*cos(th2)*sin(th1))/81129638414606681695789005144064) + sin(th3)*(cos(th1)*cos(th2) - (4967757600021511*sin(th1)*sin(th2))/81129638414606681695789005144064))*((7071*sin(pitch)*sin(yaw))/10000 - (7071*cos(roll)*cos(yaw))/10000 + (7071*cos(pitch)*sin(roll)*sin(yaw))/10000) + (cos(th3)*((4967757600021511*cos(th1)*cos(th2))/81129638414606681695789005144064 - sin(th1)*sin(th2)) - sin(th3)*((4967757600021511*cos(th1)*sin(th2))/81129638414606681695789005144064 + cos(th2)*sin(th1)))*((7071*cos(roll)*cos(yaw))/10000 + (7071*sin(pitch)*sin(yaw))/10000 - (7071*cos(pitch)*sin(roll)*sin(yaw))/10000), (cos(yaw)*sin(roll) + cos(pitch)*cos(roll)*sin(yaw))*(cos(th2)*cos(th3) - sin(th2)*sin(th3)) - (cos(th3)*(cos(th1)*sin(th2) + (4967757600021511*cos(th2)*sin(th1))/81129638414606681695789005144064) + sin(th3)*(cos(th1)*cos(th2) - (4967757600021511*sin(th1)*sin(th2))/81129638414606681695789005144064))*((7071*sin(pitch)*sin(yaw))/10000 - (7071*cos(roll)*cos(yaw))/10000 + (7071*cos(pitch)*sin(roll)*sin(yaw))/10000) + (cos(th3)*((4967757600021511*cos(th1)*cos(th2))/81129638414606681695789005144064 - sin(th1)*sin(th2)) - sin(th3)*((4967757600021511*cos(th1)*sin(th2))/81129638414606681695789005144064 + cos(th2)*sin(th1)))*((7071*cos(roll)*cos(yaw))/10000 + (7071*sin(pitch)*sin(yaw))/10000 - (7071*cos(pitch)*sin(roll)*sin(yaw))/10000), 0; ...
%  0, 0, 0, (cos(roll)*sin(yaw) + cos(pitch)*cos(yaw)*sin(roll))*(cos(th2)*sin(th3) + cos(th3)*sin(th2) + 24678615572571482867467662723121/6582018229284824168619876730229402019930943462534319453394436096) - ((7071*sin(roll)*sin(yaw))/10000 - (7071*cos(pitch)*cos(roll)*cos(yaw))/10000)*(cos(th3)*((4967757600021511*cos(th1)*sin(th2))/81129638414606681695789005144064 + cos(th2)*sin(th1)) - (4967757600021511*cos(th1))/81129638414606681695789005144064 + sin(th3)*((4967757600021511*cos(th1)*cos(th2))/81129638414606681695789005144064 - sin(th1)*sin(th2))) + ((7071*sin(roll)*sin(yaw))/10000 - (7071*cos(pitch)*cos(roll)*cos(yaw))/10000)*((4967757600021511*sin(th1))/81129638414606681695789005144064 + cos(th3)*(cos(th1)*cos(th2) - (4967757600021511*sin(th1)*sin(th2))/81129638414606681695789005144064) - sin(th3)*(cos(th1)*sin(th2) + (4967757600021511*cos(th2)*sin(th1))/81129638414606681695789005144064)), cos(roll)*cos(yaw)*sin(pitch)*(cos(th2)*sin(th3) + cos(th3)*sin(th2) + 24678615572571482867467662723121/6582018229284824168619876730229402019930943462534319453394436096) - ((7071*cos(pitch)*cos(yaw))/10000 - (7071*cos(yaw)*sin(pitch)*sin(roll))/10000)*((4967757600021511*sin(th1))/81129638414606681695789005144064 + cos(th3)*(cos(th1)*cos(th2) - (4967757600021511*sin(th1)*sin(th2))/81129638414606681695789005144064) - sin(th3)*(cos(th1)*sin(th2) + (4967757600021511*cos(th2)*sin(th1))/81129638414606681695789005144064)) - ((7071*cos(pitch)*cos(yaw))/10000 + (7071*cos(yaw)*sin(pitch)*sin(roll))/10000)*(cos(th3)*((4967757600021511*cos(th1)*sin(th2))/81129638414606681695789005144064 + cos(th2)*sin(th1)) - (4967757600021511*cos(th1))/81129638414606681695789005144064 + sin(th3)*((4967757600021511*cos(th1)*cos(th2))/81129638414606681695789005144064 - sin(th1)*sin(th2))), ((7071*sin(pitch)*sin(yaw))/10000 - (7071*cos(roll)*cos(yaw))/10000 + (7071*cos(pitch)*sin(roll)*sin(yaw))/10000)*((4967757600021511*sin(th1))/81129638414606681695789005144064 + cos(th3)*(cos(th1)*cos(th2) - (4967757600021511*sin(th1)*sin(th2))/81129638414606681695789005144064) - sin(th3)*(cos(th1)*sin(th2) + (4967757600021511*cos(th2)*sin(th1))/81129638414606681695789005144064)) + (cos(yaw)*sin(roll) + cos(pitch)*cos(roll)*sin(yaw))*(cos(th2)*sin(th3) + cos(th3)*sin(th2) + 24678615572571482867467662723121/6582018229284824168619876730229402019930943462534319453394436096) + ((7071*cos(roll)*cos(yaw))/10000 + (7071*sin(pitch)*sin(yaw))/10000 - (7071*cos(pitch)*sin(roll)*sin(yaw))/10000)*(cos(th3)*((4967757600021511*cos(th1)*sin(th2))/81129638414606681695789005144064 + cos(th2)*sin(th1)) - (4967757600021511*cos(th1))/81129638414606681695789005144064 + sin(th3)*((4967757600021511*cos(th1)*cos(th2))/81129638414606681695789005144064 - sin(th1)*sin(th2))), ((7071*cos(yaw)*sin(pitch))/10000 + (7071*cos(roll)*sin(yaw))/10000 + (7071*cos(pitch)*cos(yaw)*sin(roll))/10000)*(cos(th3)*((4967757600021511*cos(th1)*sin(th2))/81129638414606681695789005144064 + cos(th2)*sin(th1)) - (4967757600021511*cos(th1))/81129638414606681695789005144064 + sin(th3)*((4967757600021511*cos(th1)*cos(th2))/81129638414606681695789005144064 - sin(th1)*sin(th2))) + ((7071*cos(roll)*sin(yaw))/10000 - (7071*cos(yaw)*sin(pitch))/10000 + (7071*cos(pitch)*cos(yaw)*sin(roll))/10000)*((4967757600021511*sin(th1))/81129638414606681695789005144064 + cos(th3)*(cos(th1)*cos(th2) - (4967757600021511*sin(th1)*sin(th2))/81129638414606681695789005144064) - sin(th3)*(cos(th1)*sin(th2) + (4967757600021511*cos(th2)*sin(th1))/81129638414606681695789005144064)), (sin(roll)*sin(yaw) - cos(pitch)*cos(roll)*cos(yaw))*(cos(th2)*cos(th3) - sin(th2)*sin(th3)) + (cos(th3)*(cos(th1)*sin(th2) + (4967757600021511*cos(th2)*sin(th1))/81129638414606681695789005144064) + sin(th3)*(cos(th1)*cos(th2) - (4967757600021511*sin(th1)*sin(th2))/81129638414606681695789005144064))*((7071*cos(yaw)*sin(pitch))/10000 + (7071*cos(roll)*sin(yaw))/10000 + (7071*cos(pitch)*cos(yaw)*sin(roll))/10000) + (cos(th3)*((4967757600021511*cos(th1)*cos(th2))/81129638414606681695789005144064 - sin(th1)*sin(th2)) - sin(th3)*((4967757600021511*cos(th1)*sin(th2))/81129638414606681695789005144064 + cos(th2)*sin(th1)))*((7071*cos(roll)*sin(yaw))/10000 - (7071*cos(yaw)*sin(pitch))/10000 + (7071*cos(pitch)*cos(yaw)*sin(roll))/10000), (sin(roll)*sin(yaw) - cos(pitch)*cos(roll)*cos(yaw))*(cos(th2)*cos(th3) - sin(th2)*sin(th3)) + (cos(th3)*(cos(th1)*sin(th2) + (4967757600021511*cos(th2)*sin(th1))/81129638414606681695789005144064) + sin(th3)*(cos(th1)*cos(th2) - (4967757600021511*sin(th1)*sin(th2))/81129638414606681695789005144064))*((7071*cos(yaw)*sin(pitch))/10000 + (7071*cos(roll)*sin(yaw))/10000 + (7071*cos(pitch)*cos(yaw)*sin(roll))/10000) + (cos(th3)*((4967757600021511*cos(th1)*cos(th2))/81129638414606681695789005144064 - sin(th1)*sin(th2)) - sin(th3)*((4967757600021511*cos(th1)*sin(th2))/81129638414606681695789005144064 + cos(th2)*sin(th1)))*((7071*cos(roll)*sin(yaw))/10000 - (7071*cos(yaw)*sin(pitch))/10000 + (7071*cos(pitch)*cos(yaw)*sin(roll))/10000), 0];
%% task vector
Rs1 = [((7071*cos(pitch))/10000 + (7071*sin(pitch)*sin(roll))/10000)*(cos(th3)*((4967757600021511*cos(th1)*sin(th2))/81129638414606681695789005144064 + cos(th2)*sin(th1)) - (4967757600021511*cos(th1))/81129638414606681695789005144064 + sin(th3)*((4967757600021511*cos(th1)*cos(th2))/81129638414606681695789005144064 - sin(th1)*sin(th2))) + ((7071*cos(pitch))/10000 - (7071*sin(pitch)*sin(roll))/10000)*((4967757600021511*sin(th1))/81129638414606681695789005144064 + cos(th3)*(cos(th1)*cos(th2) - (4967757600021511*sin(th1)*sin(th2))/81129638414606681695789005144064) - sin(th3)*(cos(th1)*sin(th2) + (4967757600021511*cos(th2)*sin(th1))/81129638414606681695789005144064)) - cos(roll)*sin(pitch)*(cos(th2)*sin(th3) + cos(th3)*sin(th2) + 24678615572571482867467662723121/6582018229284824168619876730229402019930943462534319453394436096); ...
 ((7071*sin(pitch)*sin(yaw))/10000 - (7071*cos(roll)*cos(yaw))/10000 + (7071*cos(pitch)*sin(roll)*sin(yaw))/10000)*((4967757600021511*sin(th1))/81129638414606681695789005144064 + cos(th3)*(cos(th1)*cos(th2) - (4967757600021511*sin(th1)*sin(th2))/81129638414606681695789005144064) - sin(th3)*(cos(th1)*sin(th2) + (4967757600021511*cos(th2)*sin(th1))/81129638414606681695789005144064)) + (cos(yaw)*sin(roll) + cos(pitch)*cos(roll)*sin(yaw))*(cos(th2)*sin(th3) + cos(th3)*sin(th2) + 24678615572571482867467662723121/6582018229284824168619876730229402019930943462534319453394436096) + ((7071*cos(roll)*cos(yaw))/10000 + (7071*sin(pitch)*sin(yaw))/10000 - (7071*cos(pitch)*sin(roll)*sin(yaw))/10000)*(cos(th3)*((4967757600021511*cos(th1)*sin(th2))/81129638414606681695789005144064 + cos(th2)*sin(th1)) - (4967757600021511*cos(th1))/81129638414606681695789005144064 + sin(th3)*((4967757600021511*cos(th1)*cos(th2))/81129638414606681695789005144064 - sin(th1)*sin(th2))); ...
 (sin(roll)*sin(yaw) - cos(pitch)*cos(roll)*cos(yaw))*(cos(th2)*sin(th3) + cos(th3)*sin(th2) + 24678615572571482867467662723121/6582018229284824168619876730229402019930943462534319453394436096) + ((7071*cos(roll)*sin(yaw))/10000 - (7071*cos(yaw)*sin(pitch))/10000 + (7071*cos(pitch)*cos(yaw)*sin(roll))/10000)*(cos(th3)*((4967757600021511*cos(th1)*sin(th2))/81129638414606681695789005144064 + cos(th2)*sin(th1)) - (4967757600021511*cos(th1))/81129638414606681695789005144064 + sin(th3)*((4967757600021511*cos(th1)*cos(th2))/81129638414606681695789005144064 - sin(th1)*sin(th2))) - ((7071*cos(yaw)*sin(pitch))/10000 + (7071*cos(roll)*sin(yaw))/10000 + (7071*cos(pitch)*cos(yaw)*sin(roll))/10000)*((4967757600021511*sin(th1))/81129638414606681695789005144064 + cos(th3)*(cos(th1)*cos(th2) - (4967757600021511*sin(th1)*sin(th2))/81129638414606681695789005144064) - sin(th3)*(cos(th1)*sin(th2) + (4967757600021511*cos(th2)*sin(th1))/81129638414606681695789005144064))];
%%
invJs1 = pinv(d_Rs1);
dRs1 = d_s1 - Rs1;
%%
q_s1 = invJs1 * dRs1;
%%
N_s1 = eye(10) - invJs1*d_Rs1;

== matlab function sl_aerialmanipulator/spherical image feature errors  ==
  data: A output; p input; error output; ps input; d_h output
function [A, error, d_h] = visualerror(p, ps)
%% get the visual error message
% cal s and s*
[m,n] = size(p);
s = (1/500)*(p - repmat([640;400],[1 n]));
s = [s; ones(1,n)];
for i=1:n
    s(:,i) = s(:,i)./norm(s(:,i));
end
st = (1/500)*(ps - repmat([640;400],[1 n]));
st = [st; ones(1,n)];
for i=1:n
    st(:,i) = st(:,i)./norm(st(:,i));
end
% cal sum of s
h = sum(s,2);
ht = sum(st,2);
% delta h 
delta_h = h - ht;
d_h = delta_h;
%% modefied delta h
namda = 2;
ht_stat = ht./norm(ht);
% error = h - ht;
error = cross(ht_stat, h) + namda*ht_stat*(ht_stat'*delta_h);
%% A for use
sk_ht = [0 -ht_stat(3) ht_stat(2);...
    ht_stat(3) 0 -ht_stat(1);...
    -ht_stat(2) ht_stat(1) 0];
A = -sk_ht + namda*(ht_stat*ht_stat');

== matlab function sl_aerialmanipulator/modified pseudo inverse jacobian matrix ==
  data: Jmain input; Jpseudo output; d_h input; Nm output; namda output
function [Jpseudo, Nm, namda] = JmainModPsuMat(Jmain, d_h)
% calculate the modified pseudo-inverse of main task jacobian matrix
% zhonghang
% 2016-12-23
%% define parametes
k = 0.1;
W1 = [eye(3) zeros([3 7]); zeros([7 3]) zeros([7 7])];
W2 = [zeros([6 6]) zeros([6 4]); zeros([4 6]) diag([1 1 1 1])];
D_H = 0.8;
D_L = 0;
%% singularity avoidance matrix
Wv = 0.1*W2;
%% calculate the main psudo inverse jacobian matrix
% calculate the dynamic penalty parameter namda
norm_dh = norm(d_h);
if norm_dh <= D_L
    namda = 1;
elseif norm_dh >= D_H
    namda = 0;
else
    namda = (D_H-norm_dh)/(D_H-D_L);
end
% calculate the modified pseduo-inverse of matrix
Jpseudo = pinv(Jmain'*Jmain + k*namda*W1.^2 + k*(1-namda)*W2.^2) * Jmain';
% Jpseudo = pinv(Jmain);
% namda = 1;
% calculate the null space of the jacobian matrix
Nm = eye(10) - Jpseudo*Jmain;

== matlab function sl_aerialmanipulator/sub task two ==
  data: q_s2 output; N_s2 output; q input; d_s2 output
function [q_s2, N_s2, d_s2] = SubTskTwoJaco(q)
%#codegen
%% calculate the Rt_I matrix
th = zeros(4,1);
th = q;
%% arm parameters
% i=1
alpha0 = 0; a0 = 0.01475;
d1 = 0.15665; theta1 = 0;
% i=2
alpha1 = pi/2; a1 = 0;
d2 = 0; theta2 = 0;
% i=3
alpha2 = 0; a2 = 0.083;
d3 = 0; theta3 = pi/2;
% i=4
alpha3 = pi/2; a3 = 0;
d4 = 0.068; theta4 = pi/2;
% mass para
m0 = 2;
m1 = 0.00907; m2 = 0.27; m3 = 0.15; m4 = 0.08;
m = m1 + m2 + m3 + m4;
%%
th1 = theta1 + th(1);
th2 = theta2 + th(2);
th3 = theta3 + th(3);
th4 = theta4 + th(4);
%% sub rotation matrix
% bse transform
Base_T =[0.7071 0.7071 0 0; ...
    -0.7071 0.7071 0 0; ...
    0 0 -1.0000 0; ...
    0 0 0 1];
% arm transform matrix
T1_0 = [cos(th1) -sin(th1) 0 a0; ...
    cos(alpha0)*sin(th1) cos(alpha0)*cos(th1) -sin(alpha0) -sin(alpha0)*d1; ...
    sin(alpha0)*sin(th1) sin(alpha0)*cos(th1) cos(alpha0) cos(alpha0)*d1; ...
    0 0 0 1];
T2_1 = [cos(th2) -sin(th2) 0 a1; ...
    cos(alpha1)*sin(th2) cos(alpha1)*cos(th2) -sin(alpha1) -sin(alpha1)*d2; ...
    sin(alpha1)*sin(th2) sin(alpha1)*cos(th2) cos(alpha1) cos(alpha1)*d2; ...
    0 0 0 1];
T3_2 = [-sin(th3) -cos(th3) 0 a2; ...
    cos(alpha2)*cos(th3) -cos(alpha2)*sin(th3) -sin(alpha2) -sin(alpha2)*d3; ...
    sin(alpha2)*cos(th3) -sin(alpha2)*sin(th3) cos(alpha2) cos(alpha2)*d3; ...
    0 0 0 1];
T4_3 = [-sin(th4) -cos(th4) 0 a3; ...
    cos(alpha3)*cos(th4) -cos(alpha3)*sin(th4) -sin(alpha3) -sin(alpha3)*d4; ...
    sin(alpha3)*cos(th4) -sin(alpha3)*sin(th4) cos(alpha3) cos(alpha3)*d4; ...
    0 0 0 1];
%% calculate Pgi
Tg1 = Base_T*T1_0; Pg1 = Tg1(1:3, 4);
Tg2 = Base_T*T1_0*T2_1; Pg2 = Tg2(1:3, 4);
Tg3 = Base_T*T1_0*T2_1*T3_2; Pg3 = Tg3(1:3, 4);
Tg4 = Base_T*T1_0*T2_1*T3_2*T4_3; Pg4 = Tg4(1:3, 4);
Pg = [Pg1 Pg2 Pg3 Pg4];
%% calculate rgi
R1_b = Tg1(1:3, 1:3); R2_b = Tg2(1:3, 1:3); R3_b = Tg3(1:3, 1:3); R4_b = Tg4(1:3, 1:3);
rg1 = (1/m) * R1_b * (m1*Pg1 + m2*Pg2 + m3*Pg3 + m4*Pg4);
rg2 = (1/m) * R2_b * (m2*Pg2 + m3*Pg3 + m4*Pg4);
rg3 = (1/m) * R3_b * (m3*Pg3 + m4*Pg4);
rg4 = (1/m) * R4_b * (m4*Pg4);
%% calculate dr_th
ez = [0 0 1]';
dr_th1 = (1/m)*(m1+m2+m3+m4)*cross(R1_b*ez, rg1);
dr_th2 = (1/m)*(m2+m3+m4)*cross(R2_b*ez, rg2);
dr_th3 = (1/m)*(m3+m4)*cross(R3_b*ez, rg3);
dr_th4 = (1/m)*(m4)*cross(R4_b*ez, rg4);
Jb_g = [dr_th1 dr_th2 dr_th3 dr_th4];
%% calculate Js2 and pseduo inverse matrix
Js2 = [zeros(3,6) Jb_g];
invJs2 = pinv(Js2);
%% calculate rCG
rCG = (1/m)*(m1*Pg1 + m2*Pg2 + m3*Pg3 + m4*Pg4);
%% task error
ez = [0 0 1]';
d_s2 = (rCG'*ez)*ez - rCG;
% d_s2 = [0 0 0.1]' - rCG;
%% calculate d_s2
q_s2 = invJs2 * d_s2;
%% calculate N_s2
N_s2 = eye(10) - invJs2 * Js2;

== matlab function sl_aerialmanipulator/sub task three ==
  data: q_s3 output; N_s3 output; q input; d_s3 output
function [q_s3, N_s3, d_s3] = SubTskThreeJaco(q)
%#codegen
%% calculate the Rt_I matrix
th = zeros(4,1);
th = q;
%%
ratio = pi/180;
th1_L = -180*ratio; th1_H = 180*ratio;
th2_L = -45*ratio; th2_H = 225*ratio;
th3_L = -135*ratio; th3_H = 135*ratio;
th4_L = -180*ratio; th4_H = 180*ratio;
%%
th_L = [th1_L th2_L th3_L th4_L]';
th_H = [th1_H th2_H th3_H th4_H]';
th_d = (th_L + th_H)/2;
%% task error
d_s3 = th_d - th;
%% Js3
Js3 = [zeros(4,6) eye(4)];
invJs3 = pinv(Js3);
%% calculate d_s2
q_s3 = invJs3 * d_s3;
%% calculate N_s2
N_s3 = eye(10) - invJs3 * Js3;

== matlab function sl_aerialmanipulator/polor to cartesian ==
  data: fy input; dy output; th input
function dy = polortocart(fy, th)
%%
dy = [sin(fy)*cos(th) sin(fy)*sin(th) cos(fy)]';
